simulink model "electrical_sys"  (R2021a)
settings: Solver=VariableStepAuto  StartTime=0.0  StopTime=30  MaxStep=0.01  RelTol=1e-3
libraries: spsSeriesRLCBranchLib x4, spsDCVoltageSourceLib x1, spsVoltageMeasurementLib x1, spspowerguiLib x1
settings Model: Creator=moaza  LastModifiedBy=moaza

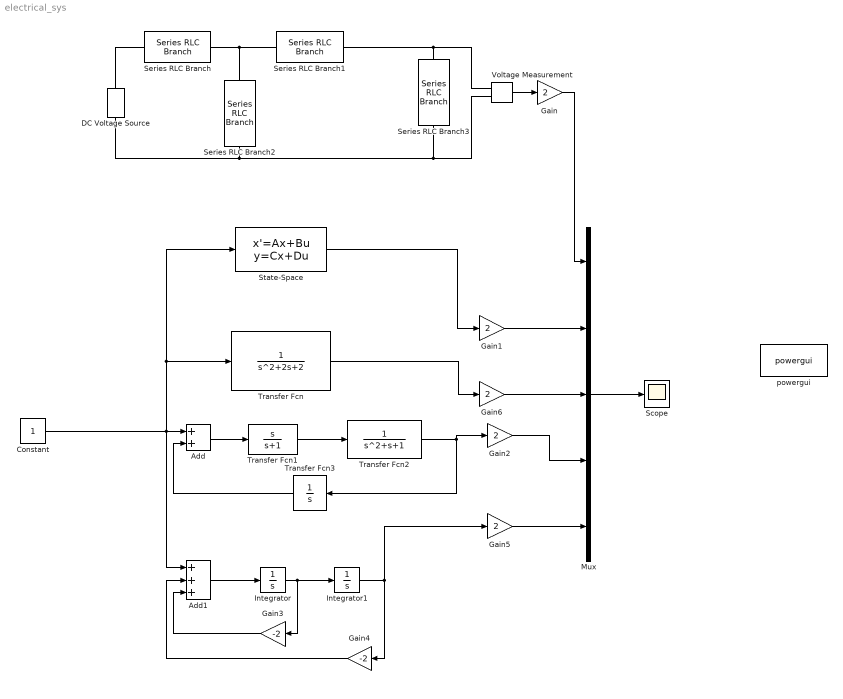
== system electrical_sys ==
  Add : Sum
  Add1 : Sum  Inputs=+++
  Constant : Constant
  DC Voltage Source : spsDCVoltageSourceLib/DC Voltage Source  Amplitude=1  Measurements=None
  Gain{,1..2,5..6} (5 alike) : Gain  Gain=2
  Gain3 : Gain  Gain=-2
  Gain4 : Gain  Gain=-2
  Integrator : Integrator
  Integrator1 : Integrator
  Mux : Mux  Inputs=5
  Scope : Scope
  Series RLC Branch : spsSeriesRLCBranchLib/Series RLC Branch  LConnTagsString=__new0  RConnTagsString=__new0  BranchType=R  Resistance=1  Inductance=1e-3  SetiL0=off  InitialCurrent=0  Capacitance=1e-6  Setx0=off  InitialVoltage=0  Measurements=None
  Series RLC Branch1 : spsSeriesRLCBranchLib/Series RLC Branch  LConnTagsString=__new0  RConnTagsString=__new0  BranchType=L  Resistance=1  Inductance=1  SetiL0=on  InitialCurrent=0  Capacitance=1e-6  Setx0=off  InitialVoltage=0  Measurements=None
  Series RLC Branch2 : spsSeriesRLCBranchLib/Series RLC Branch  LConnTagsString=__new0  RConnTagsString=__new0  BranchType=C  Resistance=1  Inductance=1  SetiL0=on  InitialCurrent=0  Capacitance=1  Setx0=on  InitialVoltage=0  Measurements=None
  Series RLC Branch3 : spsSeriesRLCBranchLib/Series RLC Branch  LConnTagsString=__new0  RConnTagsString=__new0  BranchType=R  Resistance=1  Inductance=1e-3  SetiL0=off  InitialCurrent=0  Capacitance=1e-6  Setx0=off  InitialVoltage=0  Measurements=None
  State-Space : StateSpace  A=[0 1;-2 -2]  B=[0;1]  C=[1 0]  D=0  InitialCondition=0
  Transfer Fcn : TransferFcn  Denominator=[1 2 2]
  Transfer Fcn1 : TransferFcn  Numerator=[1 0]  Denominator=[1 1]
  Transfer Fcn2 : TransferFcn  Denominator=[1 1 1]
  Transfer Fcn3 : TransferFcn  Denominator=[1 0]
  Voltage Measurement : spsVoltageMeasurementLib/Voltage Measurement  PhasorSimulation=off  OutputType=Complex  PSBequivalent=0
  powergui : spspowerguiLib/powergui  Priority=1  SimulationMode=Continuous  SampleTime=50e-6  frequency=60  Iterations=50  frequencyindice=0  Pbase=100e6  ErrMax=1e-4  UnitsV=kV  UnitsW=MW  buscounter=0  FunctionMessages=off  echomessages=off  EnableUseOfTLC=off  CurrentSourceSwitches=off  DisableSnubberDevices=off  DisableRonSwitches=off  DisableVfSwitches=off  DisplayEquations=off  AutomaticDiscreteSolvers=off  SolverType=Tustin/Backward Euler (TBE)  Interpol=off  ExternalGateDelay=off  methode=off  Ts=100  x0status=blocks  SPID=on  SwTol=0  HookPort=off  NonlinearTolerance=1e-4  nMaxIteration=100  ContinueOnMaxIteration=off  RestoreLinks=warning  ResistiveCurrentMeasurement=off  Frange=[0:2:500]  Ylog=off  Xlog=on  ShowGrid=off  save=off  variable=ZData  structure=0  ZoomFFT=off  StartTime=0.0  cycles=1  DisplayStyle=1  fundamental=60  FreqAxis=off  MaxFrequency=1000  frequencyindicesteady=1  RmsSteady=1  display=off
  wires:
  Voltage Measurement/1 -> Gain/1
  Constant/1 -> State-Space/1, Transfer Fcn/1, Add1/1, Add/1
  State-Space/1 -> Gain1/1
  Mux/1 -> Scope/1
  Gain1/1 -> Mux/2
  Gain/1 -> Mux/1
  Transfer Fcn/1 -> Gain6/1
  Add/1 -> Transfer Fcn1/1
  Transfer Fcn1/1 -> Transfer Fcn2/1
  Transfer Fcn2/1 -> Gain2/1, Transfer Fcn3/1
  Transfer Fcn3/1 -> Add/2
  Gain2/1 -> Mux/4
  Add1/1 -> Integrator/1
  Integrator/1 -> Integrator1/1, Gain3/1
  Gain3/1 -> Add1/3
  Integrator1/1 -> Gain5/1, Gain4/1
  Gain4/1 -> Add1/2
  Gain5/1 -> Mux/5
  Gain6/1 -> Mux/3
  connections:
  Series RLC Branch1/LConn1 -- Series RLC Branch/RConn1 -- Series RLC Branch2/LConn1
  Series RLC Branch1/RConn1 -- Voltage Measurement/LConn1 -- Series RLC Branch3/LConn1
  Series RLC Branch3/RConn1 -- Voltage Measurement/LConn2 -- DC Voltage Source/LConn1 -- Series RLC Branch2/RConn1
  DC Voltage Source/RConn1 -- Series RLC Branch/LConn1
